simulink model "sim_sistema_2_observador_tf"  (Simulink 7.5)
settings: Solver=ode3  StartTime=0.0  StopTime=6  FixedStep=1e-4  RelTol=1e-3
values from neighbouring files (symbols this model uses):
  A = [0 1 0;0 0 1;-6 -11 -6;]    [exemplo10_8_b.m]
  B = [0; 0; 1]    [exemplo10_8_b.m]
  K = acker(A,B,J)    [exemplo10_8_b.m]
undefined symbols (not defined in the file or in its folder): den, num
settings Model: Creator=taniel.franklin  LastModifiedBy=taniel.franklin

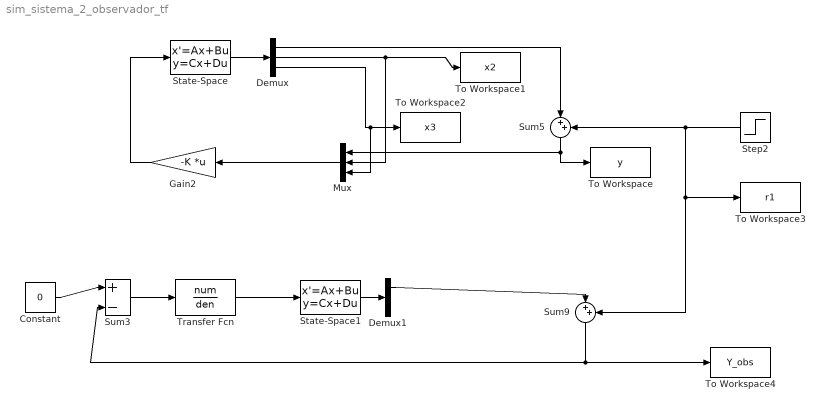
== system sim_sistema_2_observador_tf ==
  Constant : Constant  Value=0  OutDataType=fixdt(1, 16)  OutScaling=2^0
  Demux : Demux  Outputs=3
  Demux1 : Demux  Outputs=3
  Gain2 : Gain  Gain=-K  Multiplication=Matrix(K*u)  ParameterDataType=fixdt(1, 16)  ParameterScaling=2^0  OutDataType=fixdt(1, 16)  OutScaling=2^0
  Mux : Mux  Inputs=3
  State-Space : StateSpace  A=A  B=B  C=eye(3)  D=[0;0;0]
  State-Space1 : StateSpace  A=A  B=B  C=eye(3)  D=[0;0;0]
  Step2 : Step  Time=0.5  After=0.5  SampleTime=0
  Sum3 : Sum  Inputs=|+-  OutDataType=fixdt(1, 16)  OutScaling=2^0
  Sum5 : Sum  Inputs=|++  OutDataType=fixdt(1, 16)  OutScaling=2^0
  Sum9 : Sum  Inputs=|++  OutDataType=fixdt(1, 16)  OutScaling=2^0
  To Workspace : ToWorkspace  VariableName=y  SampleTime=-1  SaveFormat=Structure With Time
  To Workspace1 : ToWorkspace  VariableName=x2  SampleTime=-1  SaveFormat=Structure With Time
  To Workspace2 : ToWorkspace  VariableName=x3  SampleTime=-1  SaveFormat=Structure With Time
  To Workspace3 : ToWorkspace  VariableName=r1  SampleTime=-1  SaveFormat=Structure With Time
  To Workspace4 : ToWorkspace  VariableName=Y_obs  SampleTime=-1  SaveFormat=Structure With Time
  Transfer Fcn : TransferFcn  Numerator=num  Denominator=den
  wires:
  State-Space/1 -> Demux/1
  Demux/2 -> To Workspace1/1, Mux/2
  Demux/3 -> To Workspace2/1, Mux/3
  Gain2/1 -> State-Space/1
  Demux/1 -> Sum5/1
  State-Space1/1 -> Demux1/1
  Sum5/1 -> To Workspace/1, Mux/1
  Step2/1 -> Sum5/2, Sum9/2, To Workspace3/1
  Demux1/1 -> Sum9/1
  Sum9/1 -> Sum3/2, To Workspace4/1
  Mux/1 -> Gain2/1
  Sum3/1 -> Transfer Fcn/1
  Constant/1 -> Sum3/1
  Transfer Fcn/1 -> State-Space1/1
